simulink model "Buck_Converter"  (R2022b)
settings: Solver=VariableStepAuto  StartTime=0.0  StopTime=0.05  RelTol=1e-3
libraries: spsSeriesRLCBranchLib x3, spsDiodeLib x1, spsMosfetLib x1, spsMultimeterLib x1, spsRMSLib x1, spsDCVoltageSourceLib x1, sps_lib x1
settings Model: Creator=Biplov Jha  LastModifiedBy=Biplov Jha

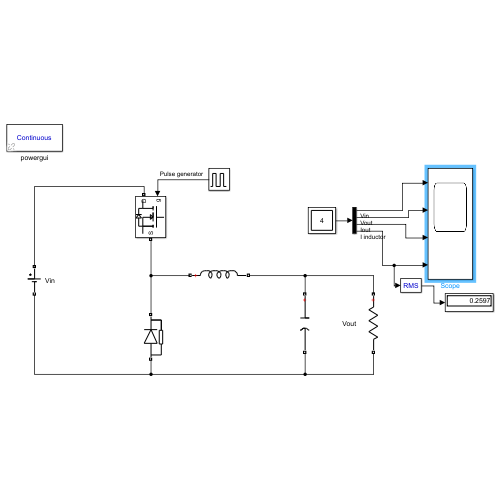
[thumbnail: Simulink's stored preview of the top-level diagram]
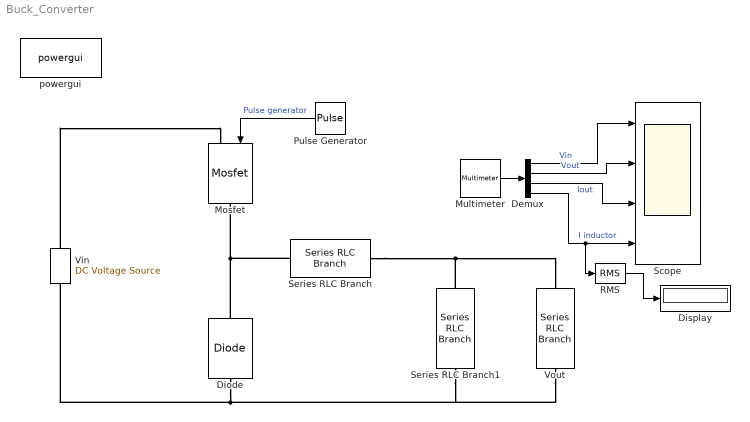
== system Buck_Converter ==
  Demux : Demux
  Diode : spsDiodeLib/Diode  Ron=0.001  Lon=0  Vf=0.8  IC=0  UseSnubber=0  Rs=500  Cs=250e-9  Measurements=off
  Display : Display
  Mosfet : spsMosfetLib/Mosfet  Ron=0.1  Lon=0  Rd=0.01  Vfd=0  IC=0  Rs=1e5  Cs=inf  Measurements=off
  Multimeter : spsMultimeterLib/Multimeter  L=4  sel=[2 1 4 3]  yselected={}  Gain=[1 1 1 1]  OutputType=Complex  PlotAtSimulationStop=off  PhasorSimulation=off
  Pulse Generator : DiscretePulseGenerator  PulseType=Time based  Period=1/(300e3)  PulseWidth=51.626
  RMS : spsRMSLib/RMS  TrueRMS=on  Freq=300e3  RMSInit=120  Ts=0
  Scope : Scope  NumInputPorts=4
  Series RLC Branch : spsSeriesRLCBranchLib/Series RLC Branch  LConnTagsString=__new0  RConnTagsString=__new0  BranchType=L  Resistance=1  Inductance=22e-6  SetiL0=off  InitialCurrent=0  Capacitance=1e-6  Setx0=off  InitialVoltage=0  Measurements=Branch current
  Series RLC Branch1 : spsSeriesRLCBranchLib/Series RLC Branch  LConnTagsString=__new0  RConnTagsString=__new0  BranchType=C  Resistance=1  Inductance=1e-3  SetiL0=off  InitialCurrent=0  Capacitance=22e-6  Setx0=off  InitialVoltage=0  Measurements=None
  Vin : spsDCVoltageSourceLib/DC Voltage Source  Amplitude=24  Measurements=Voltage
  Vout : spsSeriesRLCBranchLib/Series RLC Branch  LConnTagsString=__new0  RConnTagsString=__new0  BranchType=R  Resistance=100  Inductance=1e-3  SetiL0=off  InitialCurrent=0  Capacitance=1e-6  Setx0=off  InitialVoltage=0  Measurements=Branch voltage and current
  powergui : sps_lib/powergui  Priority=1  SimulationMode=Continuous  SampleTime=50e-6  frequency=60  Iterations=50  frequencyindice=0  Pbase=100e6  ErrMax=1e-4  UnitsV=kV  UnitsW=MW  buscounter=0  FunctionMessages=off  echomessages=off  EnableUseOfTLC=off  CurrentSourceSwitches=off  DisableSnubberDevices=off  DisableRonSwitches=off  DisableVfSwitches=off  DisplayEquations=off  AutomaticDiscreteSolvers=off  SolverType=Tustin/Backward Euler (TBE)  Interpol=off  ExternalGateDelay=off  methode=off  Ts=100  x0status=blocks  SPID=on  SwTol=0  HookPort=off  NonlinearTolerance=1e-4  nMaxIteration=100  ContinueOnMaxIteration=off  RestoreLinks=warning  ResistiveCurrentMeasurement=off  Frange=[0:2:500]  Ylog=off  Xlog=on  ShowGrid=off  save=off  variable=ZData  structure=0  ZoomFFT=off  StartTime=0.0  cycles=1  DisplayStyle=1  fundamental=60  FreqAxis=off  MaxFrequency=1000  frequencyindicesteady=1  RmsSteady=1  display=off
  wires:
  Pulse Generator/1 -> Mosfet/1  "Pulse generator"
  Multimeter/1 -> Demux/1
  Demux/1 -> Scope/1  "Vin"
  Demux/2 -> Scope/2  "Vout"
  Demux/3 -> Scope/3  "Iout"
  Demux/4 -> RMS/1, Scope/4  "I inductor"
  RMS/1 -> Display/1
  connections:
  Vin/RConn1 -- Mosfet/LConn1
  Diode/RConn1 -- Series RLC Branch/LConn1 -- Mosfet/RConn1
  Diode/LConn1 -- Series RLC Branch1/RConn1 -- Vout/RConn1 -- Vin/LConn1
  Series RLC Branch/RConn1 -- Series RLC Branch1/LConn1 -- Vout/LConn1
